simulink model "AMR_OperationModeSelector_24a"  (R2024a)
settings: configuration reference "SharedConfig" (kept outside this file)
settings Model: DataDictionary=configuration_dictionary.sldd  Creator=matlab.cut  LastModifiedBy=matlab.cut
settings ConfigSetRef: SourceName=SharedConfig

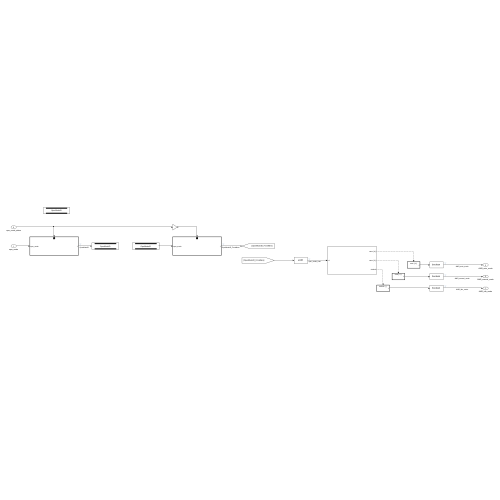
[thumbnail: Simulink's stored preview of the top-level diagram]
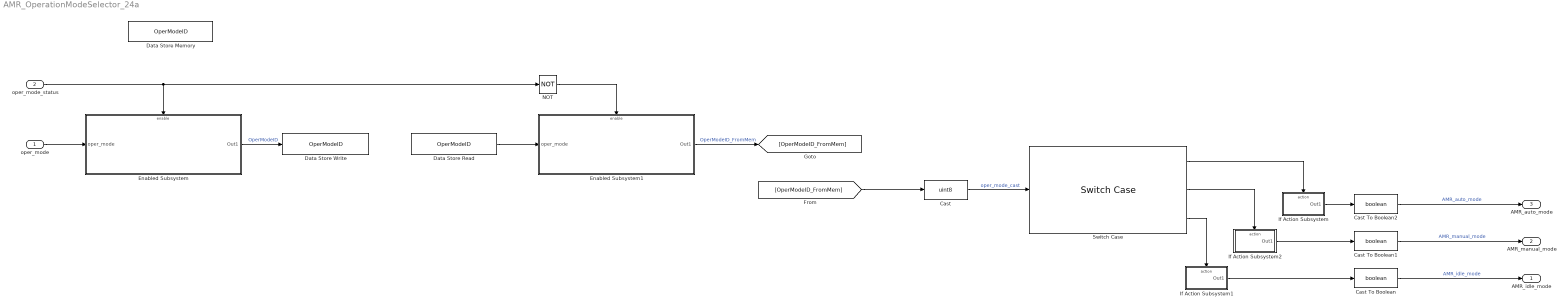
== system AMR_OperationModeSelector_24a ==
  oper_mode : Inport
  oper_mode_status : Inport  Port=2  OutDataTypeStr=boolean
  Cast : DataTypeConversion  OutDataTypeStr=uint8  SaturateOnIntegerOverflow=off  RndMeth=Floor
  Cast To Boolean : DataTypeConversion  OutDataTypeStr=boolean  SaturateOnIntegerOverflow=off  RndMeth=Floor
  Cast To Boolean1 : DataTypeConversion  OutDataTypeStr=boolean  SaturateOnIntegerOverflow=off  RndMeth=Floor
  Cast To Boolean2 : DataTypeConversion  OutDataTypeStr=boolean  SaturateOnIntegerOverflow=off  RndMeth=Floor
  Data Store Memory : DataStoreMemory  DataStoreName=OperModeID  WriteAfterWriteMsg=warning  ShowAdditionalParam=off
  Data Store Read : DataStoreRead  DataStoreName=OperModeID  DataStoreElements=OperModeID  IndexOptions=Index vector (dialog)  Indices=1  OutputSizes=1
  Data Store Write : DataStoreWrite  DataStoreName=OperModeID  DataStoreElements=OperModeID  IndexOptions=Index vector (dialog)  Indices=1  OutputSizes=1
  Enabled Subsystem : Subsystem  TreatAsAtomicUnit=on
  Enabled Subsystem1 : Subsystem  TreatAsAtomicUnit=on
  If Action Subsystem : Subsystem  TreatAsAtomicUnit=on
  If Action Subsystem1 : Subsystem  TreatAsAtomicUnit=on
  If Action Subsystem2 : Subsystem  TreatAsAtomicUnit=on
  NOT : Logic  Operator=NOT  IconShape=distinctive  AllPortsSameDT=off  OutDataTypeStr=boolean
  Switch Case : SwitchCase  CaseConditions={4,2}
  AMR_idle_mode : Outport  OutDataTypeStr=boolean
  AMR_manual_mode : Outport  Port=2  OutDataTypeStr=boolean
  AMR_auto_mode : Outport  Port=3  OutDataTypeStr=boolean
  wires:
  oper_mode/1 -> Enabled Subsystem/1(oper_mode)
  Cast/1 -> Switch Case/1  "oper_mode_cast"
  [OperModeID_FromMem] -> Cast/1
  Data Store Read/1 -> Enabled Subsystem1/1(oper_mode)
  oper_mode_status/1 -> Enabled Subsystem/Enable, NOT/1
  Enabled Subsystem1/1(Out1) -> [OperModeID_FromMem]  "OperModeID_FromMem"
  Enabled Subsystem/1(Out1) -> Data Store Write/1  "OperModeID"
  If Action Subsystem1/1(Out1) -> Cast To Boolean/1
  If Action Subsystem/1(Out1) -> Cast To Boolean2/1
  Cast To Boolean/1 -> AMR_idle_mode/1  "AMR_idle_mode"
  Cast To Boolean2/1 -> AMR_auto_mode/1  "AMR_auto_mode"
  Cast To Boolean1/1 -> AMR_manual_mode/1  "AMR_manual_mode"
  If Action Subsystem2/1(Out1) -> Cast To Boolean1/1
  Switch Case/1 -> If Action Subsystem/Action
  Switch Case/3 -> If Action Subsystem1/Action
  Switch Case/2 -> If Action Subsystem2/Action
  NOT/1 -> Enabled Subsystem1/Enable

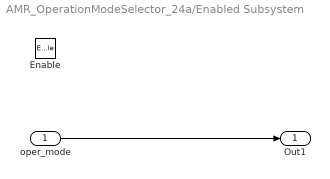
== system AMR_OperationModeSelector_24a/Enabled Subsystem ==
  oper_mode : Inport
  Enable : EnablePort
  Out1 : Outport
  wires:
  oper_mode/1 -> Out1/1

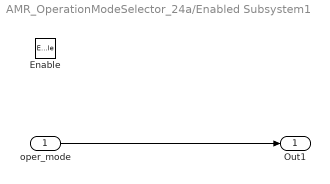
== system AMR_OperationModeSelector_24a/Enabled Subsystem1 ==
  oper_mode : Inport
  Enable : EnablePort
  Out1 : Outport  InitialOutput=0
  wires:
  oper_mode/1 -> Out1/1

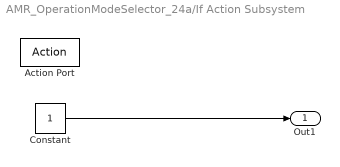
== system AMR_OperationModeSelector_24a/If Action Subsystem ==
  Action Port : ActionPort  ActionPortLabel=case [ 4 ]:
  Constant : Constant
  Out1 : Outport  OutputWhenDisabled=reset  InitialOutput=0
  wires:
  Constant/1 -> Out1/1

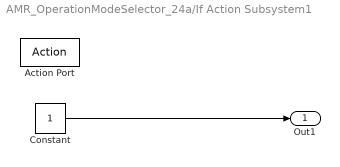
== system AMR_OperationModeSelector_24a/If Action Subsystem1 ==
  Action Port : ActionPort  ActionPortLabel=default:
  Constant : Constant
  Out1 : Outport  OutputWhenDisabled=reset  InitialOutput=0
  wires:
  Constant/1 -> Out1/1

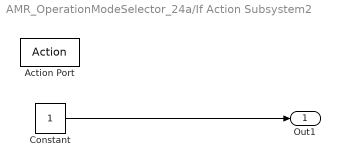
== system AMR_OperationModeSelector_24a/If Action Subsystem2 ==
  Action Port : ActionPort  ActionPortLabel=case [ 2 ]:
  Constant : Constant
  Out1 : Outport  OutputWhenDisabled=reset  InitialOutput=0
  wires:
  Constant/1 -> Out1/1
